simulink subsystem "Zw"  (R2022a)
settings: Solver=VariableStepAuto  StartTime=0.0  StopTime=10.0  RelTol=1e-3
libraries: fl_lib x200
settings Model: Creator=mmarq  LastModifiedBy=mmarq

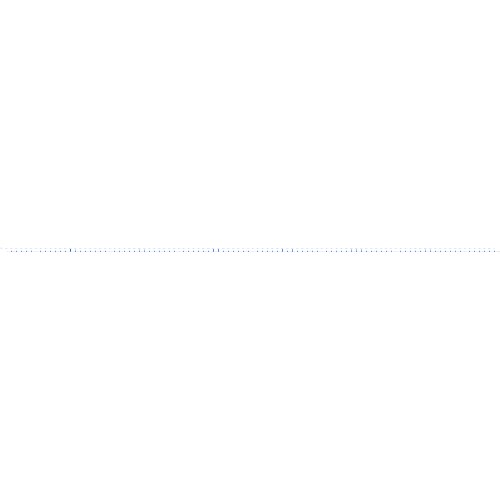
[thumbnail: Simulink's stored preview of the top-level diagram]
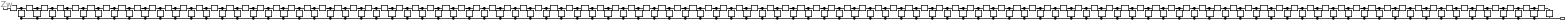
== system Zw ==
  C{1..100} (100 alike) : fl_lib/Electrical/Electrical Elements/Capacitor  c=10000 F  r=0 Ohm  g=0 1/Ohm  i_specify=off  i_priority=None  i=0 A  i_nominal_specify=off  i_nominal_unit=A  i_nominal_value=1  v_specify=off  v_priority=None  v=0 V  v_nominal_specify=off  v_nominal_unit=V  v_nominal_value=1  vc_specify=off  vc_priority=High  vc=0 V  vc_nominal_specify=off  vc_nominal_unit=V  vc_nominal_value=1
      settings: SourceProductBaseCode=PW,SS,VE
  R{1..100} (100 alike) : fl_lib/Electrical/Electrical Elements/Resistor  R=2e-05 Ohm  i_specify=off  i_priority=None  i=0 A  i_nominal_specify=off  i_nominal_unit=A  i_nominal_value=1  v_specify=off  v_priority=None  v=0 V  v_nominal_specify=off  v_nominal_unit=V  v_nominal_value=1
      settings: SourceProductBaseCode=PW,SS,VE
  + : PMIOPort  Side=Left
  - : PMIOPort  Port=2  Side=Left
  connections:
  C1/LConn1 -- R1/RConn1 -- R2/LConn1
  C2/LConn1 -- R2/RConn1 -- R3/LConn1
  C1/RConn1 -- C2/RConn1 -- C3/RConn1 -- C4/RConn1 -- C5/RConn1 -- C6/RConn1 -- C7/RConn1 -- C8/RConn1 -- C9/RConn1 -- C10/RConn1 -- C11/RConn1 -- C12/RConn1 -- C13/RConn1 -- C14/RConn1 -- C15/RConn1 -- C16/RConn1 -- C17/RConn1 -- C18/RConn1 -- C19/RConn1 -- C20/RConn1 -- C21/RConn1 -- C22/RConn1 -- C23/RConn1 -- C24/RConn1 -- C25/RConn1 -- C26/RConn1 -- C27/RConn1 -- C28/RConn1 -- C29/RConn1 -- C30/RConn1 -- C31/RConn1 -- C32/RConn1 -- C33/RConn1 -- C34/RConn1 -- C35/RConn1 -- C36/RConn1 -- C37/RConn1 -- C38/RConn1 -- C39/RConn1 -- C40/RConn1 -- C41/RConn1 -- C42/RConn1 -- C43/RConn1 -- C44/RConn1 -- C45/RConn1 -- C46/RConn1 -- C47/RConn1 -- C48/RConn1 -- C49/RConn1 -- C50/RConn1 -- C51/RConn1 -- C52/RConn1 -- C53/RConn1 -- C54/RConn1 -- C55/RConn1 -- C56/RConn1 -- C57/RConn1 -- C58/RConn1 -- C59/RConn1 -- C60/RConn1 -- C61/RConn1 -- C62/RConn1 -- C63/RConn1 -- C64/RConn1 -- C65/RConn1 -- C66/RConn1 -- C67/RConn1 -- C68/RConn1 -- C69/RConn1 -- C70/RConn1 -- C71/RConn1 -- C72/RConn1 -- C73/RConn1 -- C74/RConn1 -- C75/RConn1 -- C76/RConn1 -- C77/RConn1 -- C78/RConn1 -- C79/RConn1 -- C80/RConn1 -- C81/RConn1 -- C82/RConn1 -- C83/RConn1 -- C84/RConn1 -- C85/RConn1 -- C86/RConn1 -- C87/RConn1 -- C88/RConn1 -- C89/RConn1 -- C90/RConn1 -- C91/RConn1 -- C92/RConn1 -- C93/RConn1 -- C94/RConn1 -- C95/RConn1 -- C96/RConn1 -- C97/RConn1 -- C98/RConn1 -- C99/RConn1 -- C100/RConn1 -- -/RConn1
  C3/LConn1 -- R3/RConn1 -- R4/LConn1
  C4/LConn1 -- R4/RConn1 -- R5/LConn1
  C5/LConn1 -- R5/RConn1 -- R6/LConn1
  C6/LConn1 -- R6/RConn1 -- R7/LConn1
  C7/LConn1 -- R7/RConn1 -- R8/LConn1
  C8/LConn1 -- R8/RConn1 -- R9/LConn1
  C9/LConn1 -- R9/RConn1 -- R10/LConn1
  C10/LConn1 -- R10/RConn1 -- R11/LConn1
  C11/LConn1 -- R11/RConn1 -- R12/LConn1
  C12/LConn1 -- R12/RConn1 -- R13/LConn1
  C13/LConn1 -- R13/RConn1 -- R14/LConn1
  C14/LConn1 -- R14/RConn1 -- R15/LConn1
  C15/LConn1 -- R15/RConn1 -- R16/LConn1
  C16/LConn1 -- R16/RConn1 -- R17/LConn1
  C17/LConn1 -- R17/RConn1 -- R18/LConn1
  C18/LConn1 -- R18/RConn1 -- R19/LConn1
  C19/LConn1 -- R19/RConn1 -- R20/LConn1
  C20/LConn1 -- R20/RConn1 -- R21/LConn1
  C21/LConn1 -- R21/RConn1 -- R22/LConn1
  C22/LConn1 -- R22/RConn1 -- R23/LConn1
  C23/LConn1 -- R23/RConn1 -- R24/LConn1
  C24/LConn1 -- R24/RConn1 -- R25/LConn1
  C25/LConn1 -- R25/RConn1 -- R26/LConn1
  C26/LConn1 -- R26/RConn1 -- R27/LConn1
  C27/LConn1 -- R27/RConn1 -- R28/LConn1
  C28/LConn1 -- R28/RConn1 -- R29/LConn1
  C29/LConn1 -- R29/RConn1 -- R30/LConn1
  C30/LConn1 -- R30/RConn1 -- R31/LConn1
  C31/LConn1 -- R31/RConn1 -- R32/LConn1
  C32/LConn1 -- R32/RConn1 -- R33/LConn1
  C33/LConn1 -- R33/RConn1 -- R34/LConn1
  C34/LConn1 -- R34/RConn1 -- R35/LConn1
  C35/LConn1 -- R35/RConn1 -- R36/LConn1
  C36/LConn1 -- R36/RConn1 -- R37/LConn1
  C37/LConn1 -- R37/RConn1 -- R38/LConn1
  C38/LConn1 -- R38/RConn1 -- R39/LConn1
  C39/LConn1 -- R39/RConn1 -- R40/LConn1
  C40/LConn1 -- R40/RConn1 -- R41/LConn1
  C41/LConn1 -- R41/RConn1 -- R42/LConn1
  C42/LConn1 -- R42/RConn1 -- R43/LConn1
  C43/LConn1 -- R43/RConn1 -- R44/LConn1
  C44/LConn1 -- R44/RConn1 -- R45/LConn1
  C45/LConn1 -- R45/RConn1 -- R46/LConn1
  C46/LConn1 -- R46/RConn1 -- R47/LConn1
  C47/LConn1 -- R47/RConn1 -- R48/LConn1
  C48/LConn1 -- R48/RConn1 -- R49/LConn1
  C49/LConn1 -- R49/RConn1 -- R50/LConn1
  C50/LConn1 -- R50/RConn1 -- R51/LConn1
  C51/LConn1 -- R51/RConn1 -- R52/LConn1
  C52/LConn1 -- R52/RConn1 -- R53/LConn1
  C53/LConn1 -- R53/RConn1 -- R54/LConn1
  C54/LConn1 -- R54/RConn1 -- R55/LConn1
  C55/LConn1 -- R55/RConn1 -- R56/LConn1
  C56/LConn1 -- R56/RConn1 -- R57/LConn1
  C57/LConn1 -- R57/RConn1 -- R58/LConn1
  C58/LConn1 -- R58/RConn1 -- R59/LConn1
  C59/LConn1 -- R59/RConn1 -- R60/LConn1
  C60/LConn1 -- R60/RConn1 -- R61/LConn1
  C61/LConn1 -- R61/RConn1 -- R62/LConn1
  C62/LConn1 -- R62/RConn1 -- R63/LConn1
  C63/LConn1 -- R63/RConn1 -- R64/LConn1
  C64/LConn1 -- R64/RConn1 -- R65/LConn1
  C65/LConn1 -- R65/RConn1 -- R66/LConn1
  C66/LConn1 -- R66/RConn1 -- R67/LConn1
  C67/LConn1 -- R67/RConn1 -- R68/LConn1
  C68/LConn1 -- R68/RConn1 -- R69/LConn1
  C69/LConn1 -- R69/RConn1 -- R70/LConn1
  C70/LConn1 -- R70/RConn1 -- R71/LConn1
  C71/LConn1 -- R71/RConn1 -- R72/LConn1
  C72/LConn1 -- R72/RConn1 -- R73/LConn1
  C73/LConn1 -- R73/RConn1 -- R74/LConn1
  C74/LConn1 -- R74/RConn1 -- R75/LConn1
  C75/LConn1 -- R75/RConn1 -- R76/LConn1
  C76/LConn1 -- R76/RConn1 -- R77/LConn1
  C77/LConn1 -- R77/RConn1 -- R78/LConn1
  C78/LConn1 -- R78/RConn1 -- R79/LConn1
  C79/LConn1 -- R79/RConn1 -- R80/LConn1
  C80/LConn1 -- R80/RConn1 -- R81/LConn1
  C81/LConn1 -- R81/RConn1 -- R82/LConn1
  C82/LConn1 -- R82/RConn1 -- R83/LConn1
  C83/LConn1 -- R83/RConn1 -- R84/LConn1
  C84/LConn1 -- R84/RConn1 -- R85/LConn1
  C85/LConn1 -- R85/RConn1 -- R86/LConn1
  C86/LConn1 -- R86/RConn1 -- R87/LConn1
  C87/LConn1 -- R87/RConn1 -- R88/LConn1
  C88/LConn1 -- R88/RConn1 -- R89/LConn1
  C89/LConn1 -- R89/RConn1 -- R90/LConn1
  C90/LConn1 -- R90/RConn1 -- R91/LConn1
  C91/LConn1 -- R91/RConn1 -- R92/LConn1
  C92/LConn1 -- R92/RConn1 -- R93/LConn1
  C93/LConn1 -- R93/RConn1 -- R94/LConn1
  C94/LConn1 -- R94/RConn1 -- R95/LConn1
  C95/LConn1 -- R95/RConn1 -- R96/LConn1
  C96/LConn1 -- R96/RConn1 -- R97/LConn1
  C97/LConn1 -- R97/RConn1 -- R98/LConn1
  C98/LConn1 -- R98/RConn1 -- R99/LConn1
  C99/LConn1 -- R99/RConn1 -- R100/LConn1
  R100/RConn1 -- C100/LConn1
  +/RConn1 -- R1/LConn1
